simulink model "Simulation_Assignment_2015297"  (R2016a)
settings: Solver=VariableStepAuto  StartTime=0.0  StopTime=10.0  RelTol=1e-3
settings Model: Creator=hp  LastModifiedBy=hp

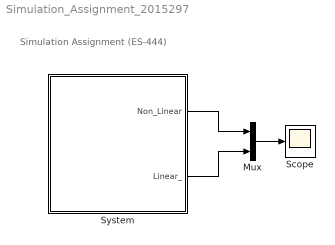
== system Simulation_Assignment_2015297 ==
  note: Simulation Assignment (ES-444)
  Mux : Mux  Inputs=2
  Scope : Scope
  System : Subsystem  mask{l=4, theta=40, g=9.8}
      mask prompts: l "Length (meter)"; theta "Theta(Degree)"; g "Gravity (m/s^2)"
  wires:
  Mux/1 -> Scope/1
  System/1(Non_Linear) -> Mux/1
  System/2(Linear_) -> Mux/2

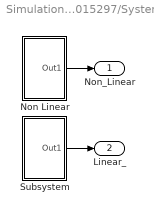
== system Simulation_Assignment_2015297/System ==
  Non Linear : Subsystem
  Subsystem : Subsystem
  Non_Linear : Outport
  Linear_ : Outport  Port=2
  wires:
  Non Linear/1(Out1) -> Non_Linear/1
  Subsystem/1(Out1) -> Linear_/1

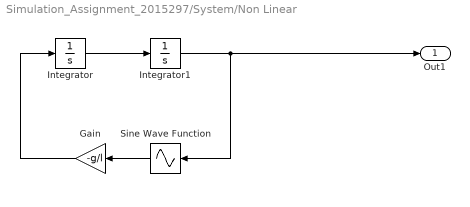
== system Simulation_Assignment_2015297/System/Non Linear ==
  Gain : Gain  Gain=-g/l
  Integrator : Integrator
  Integrator1 : Integrator  InitialCondition=theta*pi/180
  Sine Wave Function : Sin  TimeSource=Use external signal  SampleTime=0
  Out1 : Outport
  wires:
  Sine Wave Function/1 -> Gain/1
  Integrator1/1 -> Sine Wave Function/1, Out1/1
  Gain/1 -> Integrator/1
  Integrator/1 -> Integrator1/1

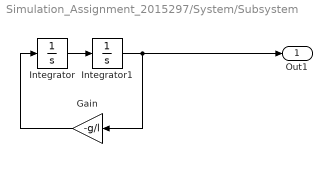
== system Simulation_Assignment_2015297/System/Subsystem ==
  Gain : Gain  Gain=-g/l
  Integrator : Integrator
  Integrator1 : Integrator  InitialCondition=theta*pi/180
  Out1 : Outport
  wires:
  Gain/1 -> Integrator/1
  Integrator1/1 -> Out1/1, Gain/1
  Integrator/1 -> Integrator1/1
